simulink model "linearizedmodel_5statespace"  (R2018b)
settings: Solver=VariableStepAuto  StartTime=0.0  StopTime=10.0  RelTol=1e-3
values from neighbouring files (symbols this model uses):
  Beq = 0.2963    [milestone2constants.m]
  Jeq = 0.01802    [milestone2constants.m]
  Kb = 2.2179e-3    (= 0.0022179)    [milestone2constants.m]
  Ke = 2.2179e-3    (= 0.0022179)    [milestone2constants.m]
  Keq = 0.74    [milestone2constants.m]
  r = 0.037    [milestone2constants.m]
  ra = 7.4    [milestone2constants.m]
  Wr = 0.18    [milestone2constants.m]
undefined symbols (not defined in the file or in its folder): s
settings Model: Creator=oliviaball  LastModifiedBy=oliviaball

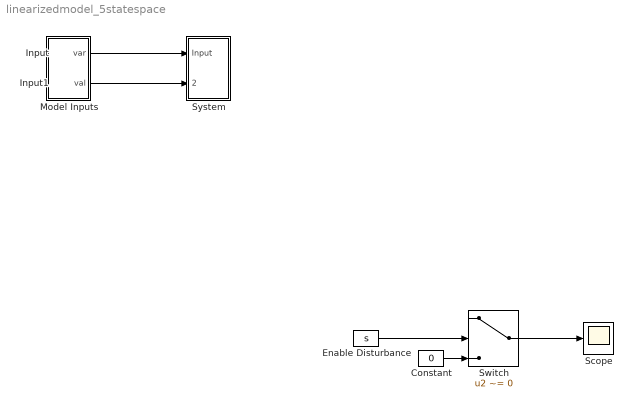
== system linearizedmodel_5statespace ==
  Input : Inport
  Input1 : Inport  Port=2
  Constant : Constant  Value=0
  Enable Disturbance : Constant  Value=s
  Model Inputs : Subsystem
  Scope : Scope
  Switch : Switch  Criteria=u2 ~= 0
  System : Subsystem
  wires:
  Model Inputs/1(var) -> System/1(Input)
  Model Inputs/2(val) -> System/2(Input1)
  Constant/1 -> Switch/3
  Enable Disturbance/1 -> Switch/2
  Switch/1 -> Scope/1

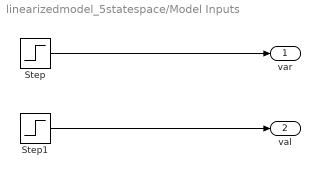
== system linearizedmodel_5statespace/Model Inputs ==
  Step : Step  SampleTime=0
  Step1 : Step  SampleTime=0
  var : Outport
  val : Outport  Port=2
  wires:
  Step1/1 -> val/1
  Step/1 -> var/1

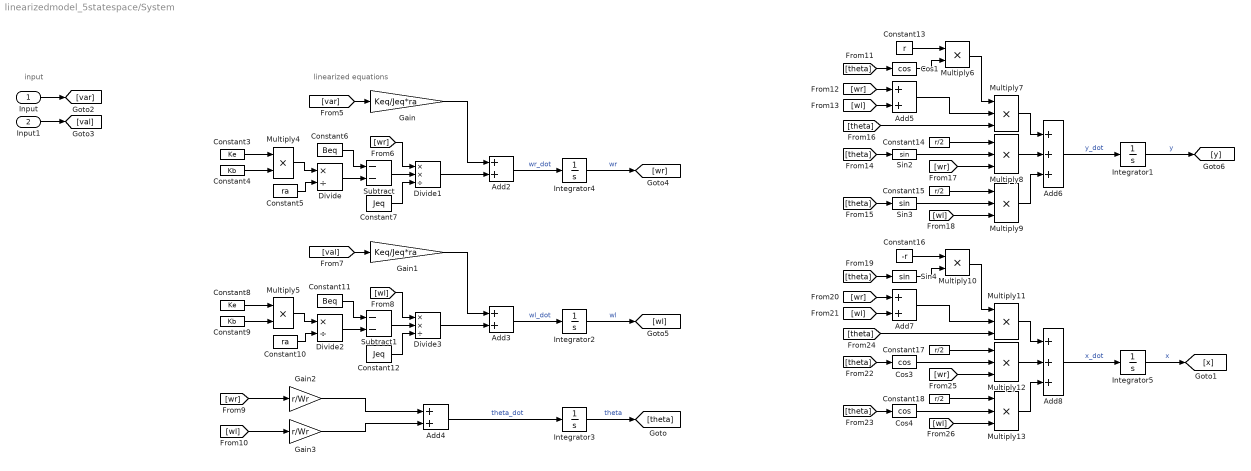
== system linearizedmodel_5statespace/System ==
  note: linearized equations
  note: input
  Input : Inport
  Input1 : Inport  Port=2
  Add{2..5,7} (5 alike) : Sum
  Add6 : Sum  Inputs=+++
  Add8 : Sum  Inputs=+++
  Constant10 : Constant  Value=ra
  Constant11 : Constant  Value=Beq
  Constant12 : Constant  Value=Jeq
  Constant13 : Constant  Value=r
  Constant{14..15,17..18} (4 alike) : Constant  Value=r/2
  Constant16 : Constant  Value=-r
  Constant3 : Constant  Value=Ke
  Constant4 : Constant  Value=Kb
  Constant5 : Constant  Value=ra
  Constant6 : Constant  Value=Beq
  Constant7 : Constant  Value=Jeq
  Constant8 : Constant  Value=Ke
  Constant9 : Constant  Value=Kb
  Cos1 : Trigonometry  Operator=cos
  Cos3 : Trigonometry  Operator=cos
  Cos4 : Trigonometry  Operator=cos
  Divide : Product  Inputs=*/
  Divide1 : Product  Inputs=**/
  Divide2 : Product  Inputs=*/
  Divide3 : Product  Inputs=**/
  Gain : Gain  Gain=Keq/Jeq*ra
  Gain1 : Gain  Gain=Keq/Jeq*ra
  Gain2 : Gain  Gain=r/Wr
  Gain3 : Gain  Gain=r/Wr
  Integrator{1..5} (5 alike) : Integrator
  Multiply{4..6,10} (4 alike) : Product
  Multiply{7..9,11..13} (6 alike) : Product  Inputs=3
  Sin2 : Trigonometry
  Sin3 : Trigonometry
  Sin4 : Trigonometry
  Subtract : Sum  Inputs=--
  Subtract1 : Sum  Inputs=--
  wires:
  [theta] -> Sin4/1
  Sin4/1 -> Multiply10/2
  Multiply9/1 -> Add6/3
  [theta] -> Cos4/1
  Constant18/1 -> Multiply13/1
  Gain3/1 -> Add4/2
  [wl] -> Add7/2
  Sin3/1 -> Multiply9/2
  Multiply10/1 -> Multiply11/1
  Add7/1 -> Multiply11/2
  Multiply12/1 -> Add8/2
  [wr] -> Multiply8/3
  Multiply8/1 -> Add6/2
  [wr] -> Multiply12/3
  Add4/1 -> Integrator3/1  "theta_dot"
  Constant7/1 -> Divide1/3
  Sin2/1 -> Multiply8/2
  [theta] -> Sin2/1
  Multiply13/1 -> Add8/3
  [wl] -> Multiply9/3
  Add5/1 -> Multiply7/2
  Gain2/1 -> Add4/1
  Cos1/1 -> Multiply6/2
  [wl] -> Multiply13/3
  [wr] -> Gain2/1
  Constant5/1 -> Divide/2
  [wr] -> Add5/1
  Cos3/1 -> Multiply12/2
  [theta] -> Cos3/1
  Multiply7/1 -> Add6/1
  [wl] -> Add5/2
  Constant12/1 -> Divide3/3
  Add2/1 -> Integrator4/1  "wr_dot"
  Gain/1 -> Add2/1
  [val] -> Gain1/1
  Constant16/1 -> Multiply10/1
  Multiply11/1 -> Add8/1
  [wl] -> Gain3/1
  Constant17/1 -> Multiply12/1
  Constant13/1 -> Multiply6/1
  Divide/1 -> Subtract/2
  [wl] -> Divide3/1
  Cos4/1 -> Multiply13/2
  Constant3/1 -> Multiply4/1
  Input/1 -> [var]
  Constant9/1 -> Multiply5/2
  Multiply4/1 -> Divide/1
  Constant14/1 -> Multiply8/1
  Integrator2/1 -> [wl]  "wl"
  Divide3/1 -> Add3/2
  Add8/1 -> Integrator5/1  "x_dot"
  [theta] -> Cos1/1
  [wr] -> Divide1/1
  Integrator4/1 -> [wr]  "wr"
  Add3/1 -> Integrator2/1  "wl_dot"
  Constant4/1 -> Multiply4/2
  Divide1/1 -> Add2/2
  Integrator3/1 -> [theta]  "theta"
  [theta] -> Sin3/1
  Gain1/1 -> Add3/1
  [theta] -> Multiply11/3
  Constant10/1 -> Divide2/2
  Multiply5/1 -> Divide2/1
  Constant11/1 -> Subtract1/1
  Integrator1/1 -> [y]  "y"
  Constant15/1 -> Multiply9/1
  Divide2/1 -> Subtract1/2
  Multiply6/1 -> Multiply7/1
  Subtract/1 -> Divide1/2
  [wr] -> Add7/1
  Constant6/1 -> Subtract/1
  Input1/1 -> [val]
  Integrator5/1 -> [x]  "x"
  [var] -> Gain/1
  [theta] -> Multiply7/3
  Add6/1 -> Integrator1/1  "y_dot"
  Subtract1/1 -> Divide3/2
  Constant8/1 -> Multiply5/1
